simulink model "chap7_2sim"  (Simulink 7.7)
settings: Solver=ode45  StartTime=0.0  StopTime=3  RelTol=1e-3
settings Model: Creator=ljk  LastModifiedBy=ljk
settings DataIOCC: SignalLoggingName=sigsOut
settings DebuggingCC: SaveWithParameterizedLinksMsg=none  SignalResolutionControl=TryResolveAllWithWarning  SolverPrmCheckMsg=none  MultiTaskDSMMsg=warning  MultiTaskCondExecSysMsg=none  StrictBusMsg=None
settings HardwareCC: TargetUnknown=on
settings RTWCC: IncludeERTFirstTime=on

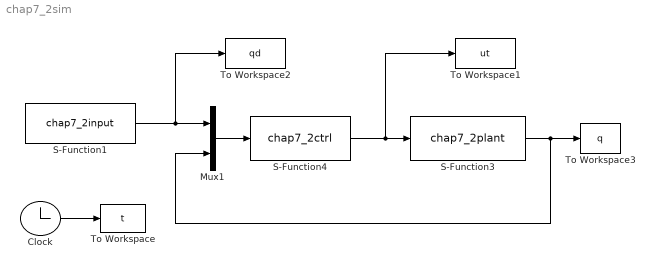
== system chap7_2sim ==
  Clock : Clock
      settings: Decimation=10
  Mux1 : Mux  Inputs=2
  S-Function1 : S-Function  FunctionName=chap7_2input  EnableBusSupport=off
  S-Function3 : S-Function  FunctionName=chap7_2plant  EnableBusSupport=off
  S-Function4 : S-Function  FunctionName=chap7_2ctrl  EnableBusSupport=off
  To Workspace : ToWorkspace  VariableName=t  SampleTime=-1  SaveFormat=Array
  To Workspace1 : ToWorkspace  VariableName=ut  SampleTime=-1  SaveFormat=Array
  To Workspace2 : ToWorkspace  VariableName=qd  SampleTime=-1  SaveFormat=Array
  To Workspace3 : ToWorkspace  VariableName=q  SampleTime=-1  SaveFormat=Array
  wires:
  S-Function4/1 -> S-Function3/1, To Workspace1/1
  S-Function3/1 -> To Workspace3/1, Mux1/2
  Mux1/1 -> S-Function4/1
  S-Function1/1 -> Mux1/1, To Workspace2/1
  Clock/1 -> To Workspace/1
